simulink model "VehicleDynamicModel"  (R2024a)
settings: Solver=VariableStepAuto  StartTime=0.0  StopTime=10.0  RelTol=1e-3
model workspace (MAT data in the model file):
  AccessoryLoad = 10
  AerodynamicDrag = 10
  DriveLineModel = 10
  FiGain = 10
  GradeForce = 10
  K = 10
  Kc = Simulink.Parameter
  Kc.Complexity = 'real'
  Kc.Dimensions = [0 0]
  Kc.DataType = 'auto'
  RollingResistance = 10
  interalResistance = 2000
  mps2kph = 3.6
  openCircuitVoltage = 560
settings Model: Creator=amtaj  LastModifiedBy=amtaj

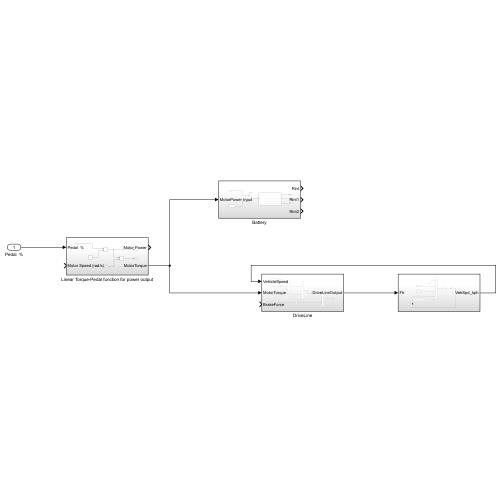
[thumbnail: Simulink's stored preview of the top-level diagram]
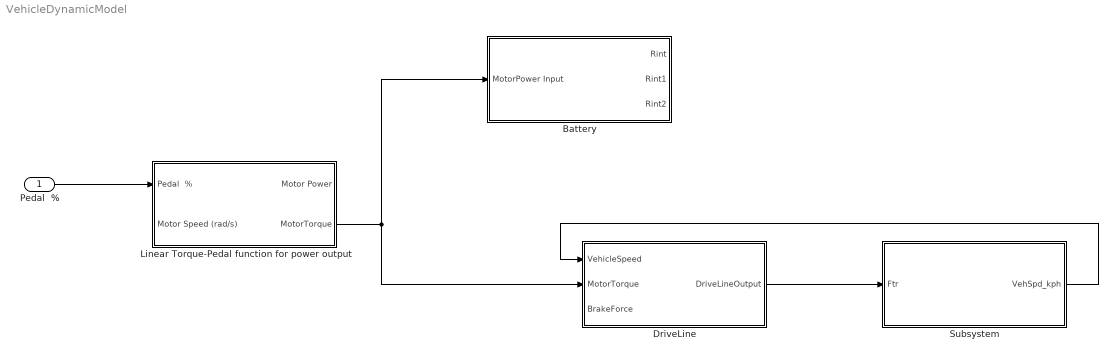
== system VehicleDynamicModel ==
  Pedal  % : Inport
  Battery : Subsystem
  DriveLine : Subsystem
  Linear Torque-Pedal function for power output : Subsystem
  Subsystem : Subsystem
  wires:
  Pedal  %/1 -> Linear Torque-Pedal function for power output/1(Pedal  %)
  DriveLine/1(DriveLineOutput) -> Subsystem/1(Ftr)
  Subsystem/1(VehSpd_kph) -> DriveLine/1(VehicleSpeed)
  Linear Torque-Pedal function for power output/2(MotorTorque) -> Battery/1(MotorPower Input), DriveLine/2(MotorTorque)

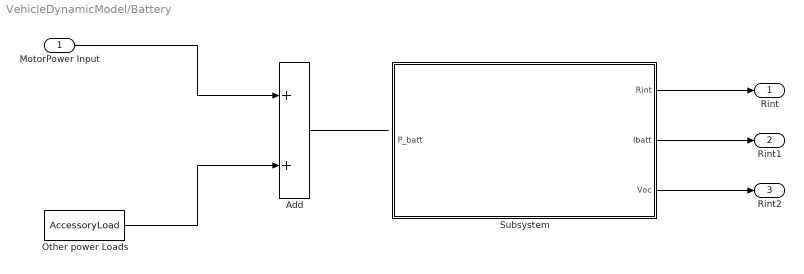
== system VehicleDynamicModel/Battery ==
  MotorPower Input : Inport
  Add : Sum
  Other power Loads : Constant  Value=AccessoryLoad
  Subsystem : Subsystem
  Rint : Outport
  Rint1 : Outport  Port=2
  Rint2 : Outport  Port=3
  wires:
  MotorPower Input/1 -> Add/1
  Other power Loads/1 -> Add/2
  Add/1 -> ?
  Subsystem/1(Rint) -> Rint/1
  Subsystem/2(Ibatt) -> Rint1/1
  Subsystem/3(Voc) -> Rint2/1

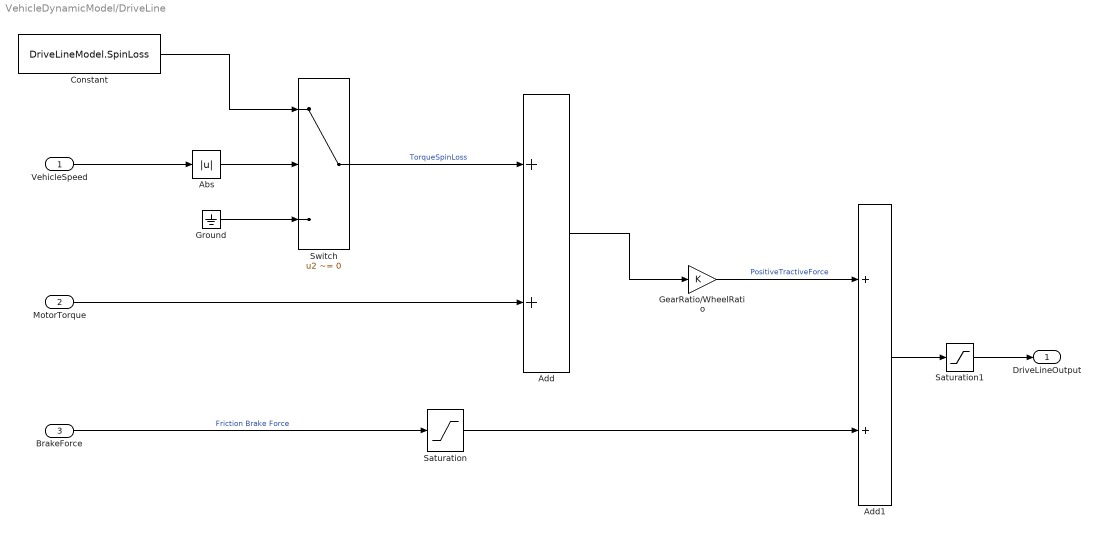
== system VehicleDynamicModel/DriveLine ==
  VehicleSpeed : Inport
  MotorTorque : Inport  Port=2
  BrakeForce : Inport  Port=3
  Abs : Abs  SaturateOnIntegerOverflow=off
  Add : Sum
  Add1 : Sum
  Constant : Constant  Value=DriveLineModel.SpinLoss
  GearRatio/WheelRatio : Gain  Gain=K
  Ground : Ground
  Saturation : Saturate
  Saturation1 : Saturate
  Switch : Switch  Criteria=u2 ~= 0  SaturateOnIntegerOverflow=off  InputSameDT=off
  DriveLineOutput : Outport
  wires:
  VehicleSpeed/1 -> Abs/1
  Abs/1 -> Switch/2
  Constant/1 -> Switch/1
  Ground/1 -> Switch/3
  MotorTorque/1 -> Add/2
  Switch/1 -> Add/1  "TorqueSpinLoss"
  Add/1 -> GearRatio/WheelRatio/1
  GearRatio/WheelRatio/1 -> Add1/1  "PositiveTractiveForce"
  BrakeForce/1 -> Saturation/1  "Friction Brake Force"
  Saturation/1 -> Add1/2
  Add1/1 -> Saturation1/1
  Saturation1/1 -> DriveLineOutput/1

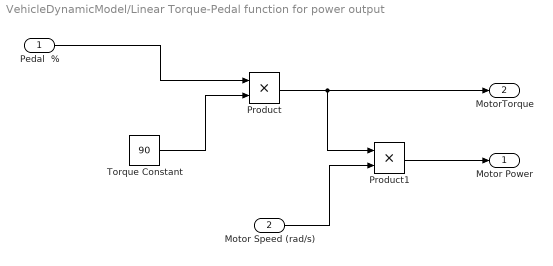
== system VehicleDynamicModel/Linear Torque-Pedal function for power output ==
  Pedal  % : Inport  OutMin=0  OutMax=1
  Motor Speed (rad/s) : Inport  Port=2
  Product : Product
  Product1 : Product
  Torque Constant : Constant  Value=90
  Motor Power : Outport
  MotorTorque : Outport  Port=2
  wires:
  Product/1 -> MotorTorque/1, Product1/1
  Torque Constant/1 -> Product/2
  Pedal  %/1 -> Product/1
  Motor Speed (rad/s)/1 -> Product1/2
  Product1/1 -> Motor Power/1

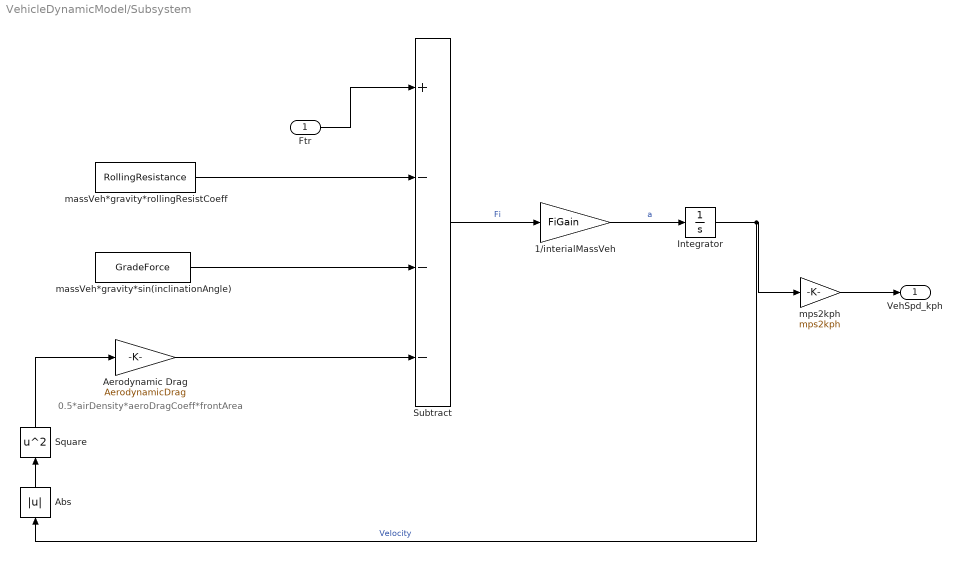
== system VehicleDynamicModel/Subsystem ==
  note: 0.5*airDensity*aeroDragCoeff*frontArea
  Ftr : Inport
  1/interialMassVeh : Gain  Gain=FiGain
  Abs : Abs  SaturateOnIntegerOverflow=off
  Aerodynamic Drag : Gain  Gain=AerodynamicDrag
  Integrator : Integrator
  Square : Math  Operator=square
  Subtract : Sum  Inputs=+---
  massVeh*gravity*rollingResistCoeff : Constant  Value=RollingResistance
  massVeh*gravity*sin(inclinationAngle) : Constant  Value=GradeForce
  mps2kph : Gain  Gain=mps2kph
  VehSpd_kph : Outport
  wires:
  Ftr/1 -> Subtract/1
  massVeh*gravity*sin(inclinationAngle)/1 -> Subtract/3
  massVeh*gravity*rollingResistCoeff/1 -> Subtract/2
  Aerodynamic Drag/1 -> Subtract/4
  Subtract/1 -> 1/interialMassVeh/1  "Fi"
  1/interialMassVeh/1 -> Integrator/1  "a"
  Integrator/1 -> Abs/1, mps2kph/1  "Velocity"
  mps2kph/1 -> VehSpd_kph/1
  Square/1 -> Aerodynamic Drag/1
  Abs/1 -> Square/1

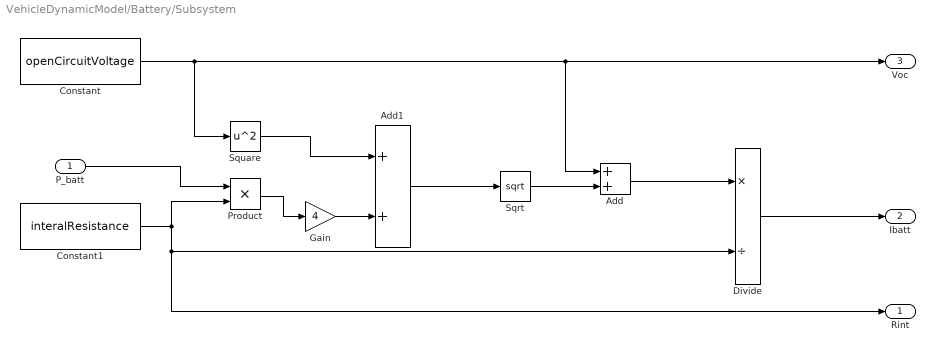
== system VehicleDynamicModel/Battery/Subsystem ==
  P_batt : Inport
  Add : Sum
  Add1 : Sum
  Constant : Constant  Value=openCircuitVoltage
  Constant1 : Constant  Value=interalResistance
  Divide : Product  Inputs=*/
  Gain : Gain  Gain=4
  Product : Product
  Sqrt : Sqrt
  Square : Math  Operator=square
  Rint : Outport
  Ibatt : Outport  Port=2
  Voc : Outport  Port=3
  wires:
  Constant/1 -> Square/1, Add/1, Voc/1
  Square/1 -> Add1/1
  Add1/1 -> Sqrt/1
  Sqrt/1 -> Add/2
  Constant1/1 -> Rint/1, Divide/2, Product/2
  P_batt/1 -> Product/1
  Product/1 -> Gain/1
  Gain/1 -> Add1/2
  Divide/1 -> Ibatt/1
  Add/1 -> Divide/1
